simulink model "PMSM_model_draft"  (R2022b)
settings: Solver=FixedStepAuto  StartTime=0.0  StopTime=Sim_Time  FixedStep=1e-4  RelTol=1e-3
values from neighbouring files (symbols this model uses):
  Pole_Pairs = 6    [PMSM_scratch_main.m]
  Position_Sensor_Offset = pi / 18    (= 0.174532925199)    [PMSM_scratch_main.m]
libraries: fl_lib x21, nesl_utility x6, ee_lib x1, simulink x1
settings Model: Creator=Administrator  LastModifiedBy=Administrator

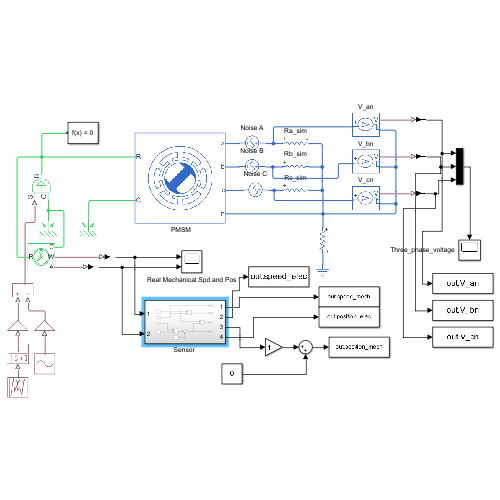
[thumbnail: Simulink's stored preview of the top-level diagram]
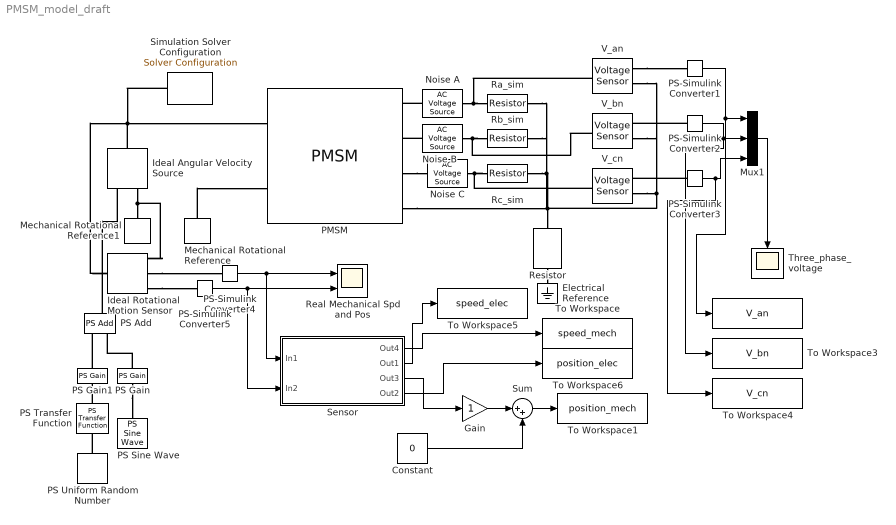
== system PMSM_model_draft ==
  "  " : ToWorkspace  VariableName=V_an  SaveFormat=Timeseries  SampleTime=-1
  " PMSM" : ee_lib/Electromechanical/Permanent Magnet/PMSM  port_option=ee.enum.threePhasePort.expanded  winding_type=ee.enum.statorconnection.wye  machine_param=ee.enum.pmsm.parameterization.constant  nPolePairs=Pole_Pairs  pmflux_param=3  pm_flux_linkage=0.03 Wb  torque_constant=0.18 N*m/A  back_emf_constant=Ke V/(rad/s)  stator_param=1  Ld=0.00025 H  Lq=0.00019 H  idVec=[-200, 0, 200] A  iqVec=[-200, 0, 200] A  LdMatrix=0.0002 * ones(3, 3) H  LqMatrix=0.0002 * ones(3, 3) H  PmMatrix=0.1 * ones(3, 3) Wb  ktMatrix=0.18 * ones(3, 3) N*m/A  keMatrix=0.18 * ones(3, 3) V/(rad/s)  L0=0.00016 H  Ls=0.0002 H  Lm=0.00002 H  Ms=0.00002 H  Rs=0.013 Ohm  zero_sequence=ee.enum.park.zerosequence.include  axes_param=2  loss_param=ee.enum.ironloss.none  losses_oc=[0, 0, 0] W  losses_sc=[0, 0, 0] W  f_losses=60 Hz  Isc_losses=95 A  J=0.01 kg*m^2  lam=0 N*m/(rad/s)  i_d_specify=off  i_d_priority=None  i_d=0 A  i_d_nominal_specify=off  i_d_nominal_unit=A  i_d_nominal_value=1  i_q_specify=off  i_q_priority=None  i_q=0 A  i_q_nominal_specify=off  i_q_nominal_unit=A  i_q_nominal_value=1  torque_specify=off  torque_priority=None  torque=0 N*m  torque_nominal_specify=off  torque_nominal_unit=N*m  torque_nominal_value=1  angular_velocity_specify=on  angular_velocity_priority=None  angular_velocity=0 rpm  angular_velocity_nominal_specify=off  angular_velocity_nominal_unit=rpm  angular_velocity_nominal_value=1  angular_position_specify=off  angular_position_priority=None  angular_position=0 deg  angular_position_nominal_specify=off  angular_position_nominal_unit=deg  angular_position_nominal_value=1  alpha=3.93e-3 1/K  alpha_flux=-0.001 1/K  Tmeas=298.15 K  stator_thermal_mass=100 J/K  rotor_thermal_mass=200 J/K  Rm_percent_rotor=90  Rd_percent_rotor=30  temperatureA_specify=off  temperatureA_priority=High  temperatureA=25 degC  temperatureA_nominal_specify=off  temperatureA_nominal_unit=degC  temperatureA_nominal_value=1  temperatureB_specify=off  temperatureB_priority=High  temperatureB=25 degC  temperatureB_nominal_specify=off  temperatureB_nominal_unit=degC  temperatureB_nominal_value=1  temperatureC_specify=off  temperatureC_priority=High  temperatureC=25 degC  temperatureC_nominal_specify=off  temperatureC_nominal_unit=degC  temperatureC_nominal_value=1  temperatureR_specify=off  temperatureR_priority=High  temperatureR=25 degC  temperatureR_nominal_specify=off  temperatureR_nominal_unit=degC  temperatureR_nominal_value=1
      settings: LogSimulationData=on  InternalSimscapePortConfiguration="{\"Bottom\":[],\"Left\":[{\"id\":\"a\",\"label\":\"a\",\"type\":\"foundation.electrical.electrical\"},{\"id\":\"b\",\"label\":\"b\",\"type\":\"foundation.electrical.electrical\"},{\"id\":\"c\",\"label\":\"c\",\"type\":\"foundation.electrical.electrical\"},{\"id\":\"n\",\"label\":\"n\",\"type\":\"foundation.electrical.electrical\"}],\"Right\":[{\"id\":\"R\",\"label\":\"R\",\"type\":\"foundation.mechanical.rotational.rotational\"},{\"id\":\"C\",\"label\":\"C\",\"type\":\"foundation.mechanical.rotational.rotational\"}],\"Top\":[]}"
  Constant : Constant  Value=0
  Electrical Reference : fl_lib/Electrical/Electrical Elements/Electrical Reference
  Gain : Gain
  Ideal Angular Velocity Source : fl_lib/Mechanical/Mechanical Sources/Ideal Angular Velocity Source
  Ideal Rotational Motion Sensor : fl_lib/Mechanical/Mechanical Sensors/Ideal Rotational Motion Sensor  reference=foundation.enum.MeasurementReference.difference  acceleration_port=false  velocity_port=true  position_port=true  wrap_angle=false  offset=0 rad
  Mechanical Rotational Reference : fl_lib/Mechanical/Rotational Elements/Mechanical Rotational Reference
  Mechanical Rotational Reference1 : fl_lib/Mechanical/Rotational Elements/Mechanical Rotational Reference
  Mux1 : Mux  Inputs=3
  Noise A : fl_lib/Electrical/Electrical Sources/AC Voltage Source  amp=.01 V  shift=0 deg  frequency=1000 Hz  omega=0 rad/s
  Noise B : fl_lib/Electrical/Electrical Sources/AC Voltage Source  amp=.01 V  shift=0 deg  frequency=1000 Hz  omega=0 rad/s
  Noise C : fl_lib/Electrical/Electrical Sources/AC Voltage Source  amp=.01 V  shift=0 deg  frequency=1000 Hz  omega=0 rad/s
  PS Add : fl_lib/Physical Signals/Functions/PS Add
  PS Gain : fl_lib/Physical Signals/Functions/PS Gain  gain=1 rad/s
  PS Gain1 : fl_lib/Physical Signals/Functions/PS Gain  gain=1 rad/s
  PS Sine Wave : fl_lib/Physical Signals/Sources/PS Sine Wave  amplitude=1  bias=0  frequency_spec=foundation.enum.frequencySpec.frequencySI  frequency_SI=5 Hz  frequency_angular=1 rad/s  phase=0 rad
      settings: InternalSimscapePortConfiguration="{\"Bottom\":[],\"Left\":[],\"Right\":[{\"id\":\"O\",\"label\":\"\",\"type\":\"output\"}],\"Top\":[]}"
  PS Transfer Function : fl_lib/Physical Signals/Linear Operators/PS Transfer Function  transfer_function_type=foundation.enum.transfer_function_type.lag  T=1 s  T1=2 s  T2=1 s  reset_method=foundation.enum.IntegratorResetSpec.None  initial_condition_spec=foundation.enum.IntegratorICSpec.Internal  y0=0
      settings: InternalSimscapePortConfiguration="{\"Bottom\":[],\"Left\":[{\"id\":\"U\",\"label\":\"\",\"type\":\"input\"}],\"Right\":[{\"id\":\"Y\",\"label\":\"\",\"type\":\"output\"}],\"Top\":[]}"
  PS Uniform Random Number : fl_lib/Physical Signals/Sources/PS Uniform Random Number  minimum=0  maximum=5  initial_seed=0  sample_time=1 ms
      settings: InternalSimscapePortConfiguration="{\"Bottom\":[],\"Left\":[],\"Right\":[{\"id\":\"Y\",\"label\":\"Y\",\"type\":\"output\"}],\"Top\":[]}"
  PS-Simulink Converter{1..5} (5 alike) : nesl_utility/PS-Simulink Converter  PhysicalDomain=network_engine_domain  SubClassName=ps_output  LeftPortType=input  RightPortType=output  PseudoPeriodic=off  Frequencies=[]  VectorFormat=1-D array  Unit=1  AffineConversion=off
  Ra_sim : fl_lib/Electrical/Electrical Elements/Resistor  R=1e10 Ohm  i_specify=off  i_priority=None  i=0 A  i_nominal_specify=off  i_nominal_unit=A  i_nominal_value=1  v_specify=off  v_priority=None  v=0 V  v_nominal_specify=off  v_nominal_unit=V  v_nominal_value=1
      settings: LogSimulationData=on
  Rb_sim : fl_lib/Electrical/Electrical Elements/Resistor  R=1e10 Ohm  i_specify=off  i_priority=None  i=0 A  i_nominal_specify=off  i_nominal_unit=A  i_nominal_value=1  v_specify=off  v_priority=None  v=0 V  v_nominal_specify=off  v_nominal_unit=V  v_nominal_value=1
  Rc_sim : fl_lib/Electrical/Electrical Elements/Resistor  R=1e10 Ohm  i_specify=off  i_priority=None  i=0 A  i_nominal_specify=off  i_nominal_unit=A  i_nominal_value=1  v_specify=off  v_priority=None  v=0 V  v_nominal_specify=off  v_nominal_unit=V  v_nominal_value=1
  Real Mechanical Spd and Pos : Scope  NumInputPorts=2
  Resistor : fl_lib/Electrical/Electrical Elements/Resistor  R=1e8 Ohm  i_specify=off  i_priority=None  i=0 A  i_nominal_specify=off  i_nominal_unit=A  i_nominal_value=1  v_specify=off  v_priority=None  v=0 V  v_nominal_specify=off  v_nominal_unit=V  v_nominal_value=1
  "Sensor " : Subsystem
  Simulation Solver Configuration : nesl_utility/Solver Configuration  PhysicalDomain=network_engine_domain  SubClassName=solver  LeftPortType=input  RightPortType=generic  Tones=[]  Harmonics=[]  SimulateNoise=off  Profile=off  UseLocalSampling=off  EnableSwitchedLinearOptims=on  FrequencyDomain=off  UseCCode=off  RelTol=0.001  AbsTol=1e-06  MinStep=1e-09  ToWorkspace=off  RevertToSquareIcSolve=off  NumHomotopyIterations=100  PhasorMode=off  PhasorModeNumHarmonics=1  ConsistencySolver=NEWTON_FTOL  IndexReductionMethod=DerivativeReplacement  DoDC=off  ResidualTolerance=1e-09  ConsistencyTolSource=GLOBAL  ConsistencyAbsTol=0.001  ConsistencyRelTol=0.001  ConsistencyTolFactor=0.001  UseLocalSolver=off  LocalSolverChoice=NE_BACKWARD_EULER_ADVANCER  ResolveIndetEquations=on  FunctionEvalNumThread=1  LocalSolverSampleTime=0.001  DoFixedCost=off  MaxNonlinIter=3  MaxModeIter=2  ComputeImpulses=off  ImpulseIterations=2  LinearAlgebra=auto  LinearAlgebraNumThread=0  EquationFormulation=NE_TIME_EF  DelaysMemoryBudget=1024  AutomaticFiltering=on  FilteringTimeConstant=0.001  PartitionStorageMethod=AS_NEEDED  PartitionMemoryBudget=1024  PartitionMethod=FAST
  Sum : Sum  Inputs=|++
  Three_phase_voltage : Scope
  To Workspace : ToWorkspace  VariableName=speed_mech  SaveFormat=Timeseries  SampleTime=-1
  To Workspace1 : ToWorkspace  VariableName=position_mech  SaveFormat=Timeseries  SampleTime=-1
  To Workspace3 : ToWorkspace  VariableName=V_bn  SaveFormat=Timeseries  SampleTime=-1
  To Workspace4 : ToWorkspace  VariableName=V_cn  SaveFormat=Timeseries  SampleTime=-1
  To Workspace5 : ToWorkspace  VariableName=speed_elec  SaveFormat=Timeseries  SampleTime=-1
  To Workspace6 : ToWorkspace  VariableName=position_elec  SaveFormat=Timeseries  SampleTime=-1
  V_an : fl_lib/Electrical/Electrical Sensors/Voltage Sensor
      settings: LogSimulationData=on
  V_bn : fl_lib/Electrical/Electrical Sensors/Voltage Sensor
      settings: LogSimulationData=on
  V_cn : fl_lib/Electrical/Electrical Sensors/Voltage Sensor
      settings: LogSimulationData=on
  wires:
  PS-Simulink Converter5/1 -> Real Mechanical Spd and Pos/2, "Sensor "/2(In2)
  PS-Simulink Converter4/1 -> Real Mechanical Spd and Pos/1, "Sensor "/1(In1)
  Mux1/1 -> Three_phase_voltage/1
  PS-Simulink Converter1/1 -> Mux1/1, "  "/1
  PS-Simulink Converter2/1 -> Mux1/2, To Workspace3/1
  PS-Simulink Converter3/1 -> To Workspace4/1, Mux1/3
  "Sensor "/1(Out4) -> To Workspace/1
  "Sensor "/2(Out1) -> To Workspace5/1
  "Sensor "/4(Out2) -> To Workspace6/1
  "Sensor "/3(Out3) -> Gain/1
  Gain/1 -> Sum/1
  Sum/1 -> To Workspace1/1
  Constant/1 -> Sum/2
  connections:
  Mechanical Rotational Reference/LConn1 -- " PMSM"/RConn2
  Ideal Angular Velocity Source/LConn1 -- Simulation Solver Configuration/RConn1 -- " PMSM"/RConn1 -- Ideal Rotational Motion Sensor/LConn1
  PS Add/RConn1 -- Ideal Angular Velocity Source/RConn1
  Ideal Angular Velocity Source/RConn2 -- Ideal Rotational Motion Sensor/RConn1 -- Mechanical Rotational Reference1/LConn1
  Ideal Rotational Motion Sensor/RConn2 -- PS-Simulink Converter4/LConn1
  Ideal Rotational Motion Sensor/RConn3 -- PS-Simulink Converter5/LConn1
  Resistor/RConn1 -- Electrical Reference/LConn1
  " PMSM"/LConn4 -- Resistor/LConn1 -- V_an/RConn2 -- V_bn/RConn2 -- V_cn/RConn2 -- Ra_sim/RConn1 -- Rb_sim/RConn1 -- Rc_sim/RConn1
  V_an/LConn1 -- Noise A/LConn1 -- Ra_sim/LConn1
  V_bn/LConn1 -- Noise B/LConn1 -- Rb_sim/LConn1
  V_cn/LConn1 -- Noise C/LConn1 -- Rc_sim/LConn1
  PS Gain/LConn1 -- PS Sine Wave/RConn1
  PS Gain/RConn1 -- PS Add/LConn2
  PS Gain1/RConn1 -- PS Add/LConn1
  PS Transfer Function/RConn1 -- PS Gain1/LConn1
  PS Uniform Random Number/RConn1 -- PS Transfer Function/LConn1
  V_an/RConn1 -- PS-Simulink Converter1/LConn1
  PS-Simulink Converter2/LConn1 -- V_bn/RConn1
  PS-Simulink Converter3/LConn1 -- V_cn/RConn1
  Noise A/RConn1 -- " PMSM"/LConn1
  Noise B/RConn1 -- " PMSM"/LConn2
  " PMSM"/LConn3 -- Noise C/RConn1

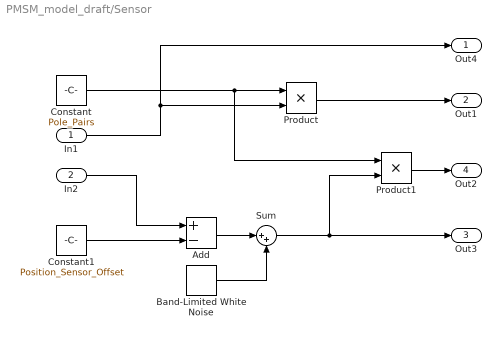
== system PMSM_model_draft/Sensor  ==
  In1 : Inport
  In2 : Inport  Port=2
  Add : Sum  Inputs=+-
  Band-Limited White Noise : simulink/Sources/Band-Limited White Noise  Cov=[1e-6]  Ts=0.001  seed=[23341]
  Constant : Constant  Value=Pole_Pairs
  Constant1 : Constant  Value=Position_Sensor_Offset
  Product : Product
  Product1 : Product
  Sum : Sum  Inputs=|++
  Out4 : Outport
  Out1 : Outport  Port=2
  Out3 : Outport  Port=3
  Out2 : Outport  Port=4
  wires:
  Product/1 -> Out1/1
  Constant1/1 -> Add/2
  In1/1 -> Out4/1, Product/2
  Constant/1 -> Product1/1, Product/1
  In2/1 -> Add/1
  Product1/1 -> Out2/1
  Add/1 -> Sum/1
  Band-Limited White Noise/1 -> Sum/2
  Sum/1 -> Out3/1, Product1/2
